simulink model "Sim43"  (R2019a)
settings: Solver=FixedStepAuto  StartTime=0.0  StopTime=10.0  FixedStep=0.0001  RelTol=1e-3
settings Model: Creator=fbleo  LastModifiedBy=fbleo

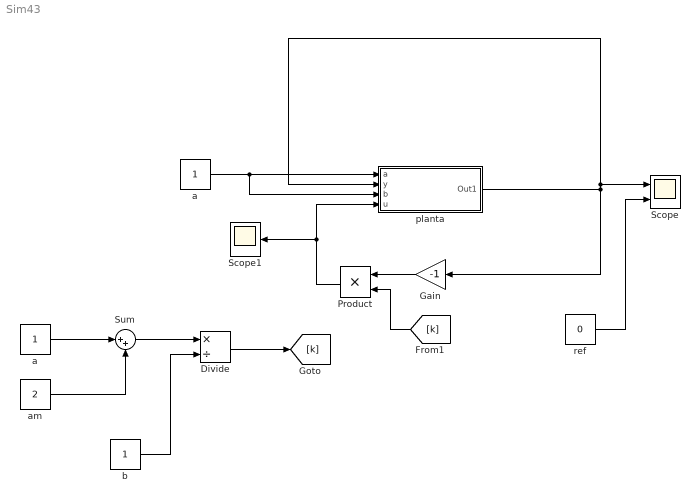
== system Sim43 ==
  Divide : Product  Inputs=*/
  Gain : Gain  Gain=-1
  Product : Product
  Scope : Scope  NumInputPorts=2
  Scope1 : Scope
  Sum : Sum  Inputs=|++
  a : Constant
  "a " : Constant
  am : Constant  Value=2
  b : Constant
  planta : Subsystem
  ref : Constant  Value=0
  wires:
  planta/1(Out1) -> planta/2(y), Scope/1, Gain/1
  a/1 -> planta/3(b), planta/1(a)
  Sum/1 -> Divide/1
  b/1 -> Divide/2
  "a "/1 -> Sum/1
  am/1 -> Sum/2
  Divide/1 -> [k]
  [k] -> Product/2
  Gain/1 -> Product/1
  Product/1 -> planta/4(u), Scope1/1
  ref/1 -> Scope/2

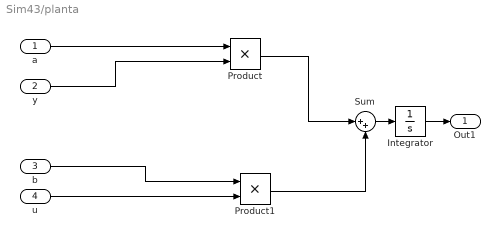
== system Sim43/planta ==
  a : Inport
  y : Inport  Port=2
  b : Inport  Port=3
  u : Inport  Port=4
  Integrator : Integrator  InitialCondition=0.5
  Product : Product
  Product1 : Product
  Sum : Sum  Inputs=|++
  Out1 : Outport
  wires:
  a/1 -> Product/1
  y/1 -> Product/2
  Product/1 -> Sum/1
  u/1 -> Product1/2
  b/1 -> Product1/1
  Product1/1 -> Sum/2
  Sum/1 -> Integrator/1
  Integrator/1 -> Out1/1
